simulink model "i2s_UART"  (R2019a)
settings: Solver=FixedStepAuto  StartTime=0.0  StopTime=inf  RelTol=1e-3
PreLoadFcn:
  | buf_size = 160
InitFcn:
  | buf_size = 160
StartFcn:
  | buf_size = 160
StopFcn:
  | audio_save_script
undefined symbols (not defined in the file or in its folder): serial
libraries: dspvision x3, instrumentlib x2, dspsnks4 x1
settings Model: Creator=HyperPC  LastModifiedBy=CIT_007
settings DataIOCC: ReturnWorkspaceOutputs=off
settings DebuggingCC: ArithmeticOperatorsInVariantConditions=warning
settings SFSimCC: SimUseLocalCustomCode=off
settings RTWCC: RTWUseLocalCustomCode=off

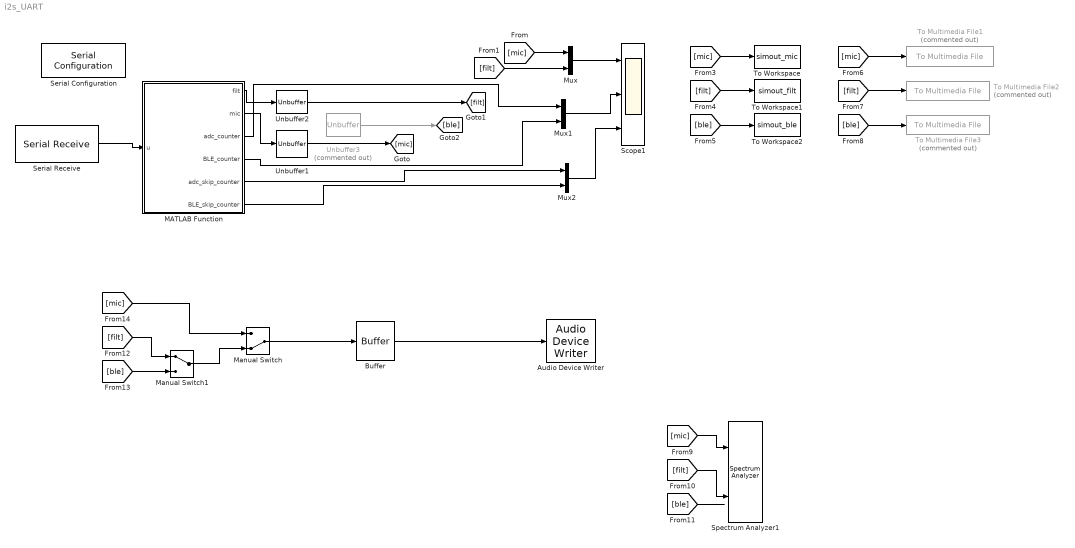
== system i2s_UART ==
  Audio Device Writer : dspsnks4/Audio Device Writer  Driver=DirectSound  Device=Default  InheritSampleRate=off  SampleRate=16000  BitDepth=16-bit integer  BufferSize=4096  NumBuffers=10  DefaultOutputChannelMapping=on  OutputChannelMapping=1:2  OutputNumUnderrunSamples=off  DriverIdx=1  DeviceWarnFlag=''
  Buffer : Buffer  N=1024  OutputFrames=off
  MATLAB Function : MATLAB Function  TreatAsAtomicUnit=on
  Manual Switch : ManualSwitch  CurrentSetting=0
  Manual Switch1 : ManualSwitch
  Mux : Mux  Inputs=2
  Mux1 : Mux  Inputs=2
  Mux2 : Mux  Inputs=2
  Scope1 : Scope  NumInputPorts=3
  Serial Configuration : instrumentlib/Serial Configuration  Priority=-200000  ComPortMenu=COM30  ComPort=COM30  ObjConstructor=serial('COM30');  BaudRate=921600  DataBits=8  Parity=none  StopBits=1  FlowControl=none  Timeout=1  ByteOrder=LittleEndian
  Serial Receive : instrumentlib/Serial Receive  ComPortMenu=COM30  ComPort=COM30  ObjConstructor=serial('COM30');  Header=)(  Terminator=<none>  DataSize="[644    1]"  DataType=int16  EnableBlockingMode=on  ActionDataUnavailable=Output custom value  CustomValue=255  SampleTime=0.02
  Spectrum Analyzer1 : SpectrumAnalyzer  NumInputPorts=2
  To Multimedia File1 : dspvision/To Multimedia File  Commented=on  outputFilename=mic.wav  streamSelection=Audio only  videoCompressor=None (uncompressed)  audioCompressor=None (uncompressed)  imagePorts=Separate color signals  fileType=WAV  audioDatatype=16-bit integer  fourcc=RGB  videoQuality=75  mj2000CompFactor=10
      settings: SourceProductName=Computer Vision Toolbox  SourceProductBaseCode=VP
  To Multimedia File2 : dspvision/To Multimedia File  Commented=on  outputFilename=mic.wav  streamSelection=Audio only  videoCompressor=None (uncompressed)  audioCompressor=None (uncompressed)  imagePorts=Separate color signals  fileType=WAV  audioDatatype=16-bit integer  fourcc=RGB  videoQuality=75  mj2000CompFactor=10
      settings: SourceProductName=Computer Vision Toolbox  SourceProductBaseCode=VP
  To Multimedia File3 : dspvision/To Multimedia File  Commented=on  outputFilename=ble.wav  streamSelection=Audio only  videoCompressor=None (uncompressed)  audioCompressor=None (uncompressed)  imagePorts=Separate color signals  fileType=WAV  audioDatatype=16-bit integer  fourcc=RGB  videoQuality=75  mj2000CompFactor=10
      settings: SourceProductName=Computer Vision Toolbox  SourceProductBaseCode=VP
  To Workspace : ToWorkspace  VariableName=simout_mic  SampleTime=1/16000
      settings: Save2DSignal=2-D array (concatenate along first dimension)
  To Workspace1 : ToWorkspace  VariableName=simout_filt  SampleTime=1/16000
      settings: Save2DSignal=2-D array (concatenate along first dimension)
  To Workspace2 : ToWorkspace  VariableName=simout_ble  SampleTime=1/16000
      settings: Save2DSignal=2-D array (concatenate along first dimension)
  Unbuffer1 : Unbuffer
  Unbuffer2 : Unbuffer
  Unbuffer3 : Unbuffer  Commented=on
  wires:
  MATLAB Function/2(mic) -> Unbuffer1/1
  MATLAB Function/1(filt) -> Unbuffer2/1
  Mux/1 -> Scope1/1
  Mux1/1 -> Scope1/2
  [ble] -> To Workspace2/1
  [filt] -> To Workspace1/1
  [mic] -> To Workspace/1
  [mic] -> To Multimedia File1/1
  [filt] -> To Multimedia File2/1
  [ble] -> To Multimedia File3/1
  [mic] -> Spectrum Analyzer1/1
  [filt] -> Spectrum Analyzer1/2
  [ble] -> ?
  [mic] -> Manual Switch/1
  [filt] -> Manual Switch1/1
  [ble] -> Manual Switch1/2
  Manual Switch1/1 -> Manual Switch/2
  Manual Switch/1 -> Buffer/1
  Serial Receive/1 -> MATLAB Function/1(u)
  Unbuffer1/1 -> [mic]
  Unbuffer2/1 -> [filt]
  Unbuffer3/1 -> [ble]
  Buffer/1 -> Audio Device Writer/1
  [mic] -> Mux/1
  [filt] -> Mux/2
  Mux2/1 -> Scope1/3
  MATLAB Function/5(adc_skip_counter) -> Mux2/1
  MATLAB Function/6(BLE_skip_counter) -> Mux2/2
  MATLAB Function/3(adc_counter) -> Mux1/1
  MATLAB Function/4(BLE_counter) -> Mux1/2

== matlab function i2s_UART/MATLAB Function ==
  data: filt output; u input; mic output [80..3200]; adc_counter output; BLE_counter output; adc_skip_counter output; BLE_skip_counter output
%function [mic, filt, ble] = fcn(u)
function [filt, mic , adc_counter, BLE_counter, adc_skip_counter, BLE_skip_counter]  = fcn(u)
persistent current_adc_frame;
persistent current_BLE_frame;

persistent total_adc_skips;
persistent total_BLE_skips;

if isempty(current_adc_frame)
    current_adc_frame = int16(0);
    current_BLE_frame = int16(0);
    total_adc_skips = int16(0);
    total_BLE_skips = int16(0);
end
    
buf_size = 320;
mic  = u(1:buf_size);
filt = u((buf_size + 1)    :(buf_size * 2));

adc_counter = (u(buf_size * 2 + 1))^16 + u(buf_size * 2 + 2);

BLE_counter = (u(buf_size * 2 + 3))^16 + u(buf_size * 2 + 4);


if adc_counter ~= (current_adc_frame+1)
    total_adc_skips = total_adc_skips + (adc_counter - current_adc_frame+1);
    adc_skip_counter = total_adc_skips;
else
    adc_skip_counter = int16(0);
end

if BLE_counter ~= (current_BLE_frame+1)
    total_BLE_skips = total_BLE_skips + (BLE_counter - current_BLE_frame+1);
    BLE_skip_counter = total_BLE_skips;
else
    BLE_skip_counter = int16(0);
end


current_adc_frame = adc_counter;
current_BLE_frame = BLE_counter;
